simulink model "sysID_model"  (R2024a)
settings: Solver=VariableStepAuto  StartTime=0.0  StopTime=T + Ttrans - Ts  RelTol=1e-3
values from neighbouring files (symbols this model uses):
  N = 100    [sysID_init.m]
  T = 15    [sysID_init.m]
  Ts = 0.002    [sysID_init.m]    (also in sysID_stiffy.m)
libraries: cstblocks x1
settings Model: Creator=dunni  LastModifiedBy=quarc_user

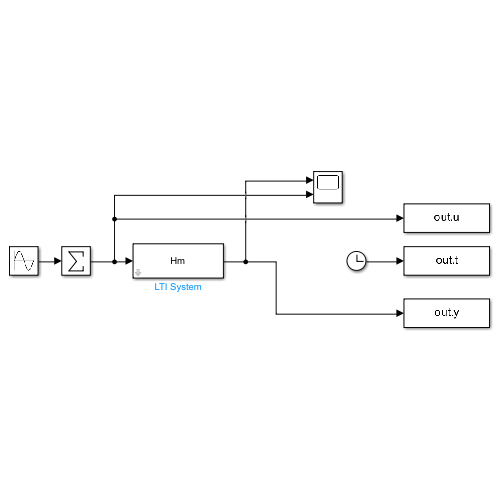
[thumbnail: Simulink's stored preview of the top-level diagram]
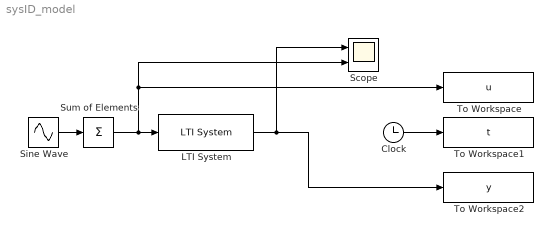
== system sysID_model ==
  Clock : Clock
  LTI System : cstblocks/LTI System  sys=Hm  IC=[]  PadeOrder=0
  Scope : Scope  NumInputPorts=2
  Sine Wave : Sin  Frequency=(1:N)*2*pi/T  Phase=rand(N,1)*2*pi  SampleTime=0
  Sum of Elements : Sum  Inputs=+
  To Workspace : ToWorkspace  VariableName=u  SampleTime=Ts
      settings: MaxDataPoints=T/Ts
  To Workspace1 : ToWorkspace  VariableName=t  SampleTime=Ts
      settings: MaxDataPoints=T/Ts
  To Workspace2 : ToWorkspace  VariableName=y  SampleTime=Ts
      settings: MaxDataPoints=T/Ts
  wires:
  Sine Wave/1 -> Sum of Elements/1
  Clock/1 -> To Workspace1/1
  Sum of Elements/1 -> LTI System/1, To Workspace/1, Scope/2
  LTI System/1 -> Scope/1, To Workspace2/1
